simulink model "RobotSim_v0p1"  (R2025b)
settings: Solver=FixedStepAuto  StartTime=0.0  StopTime=99999  RelTol=1e-3
values from neighbouring files (symbols this model uses):
  maxSteeringVel = 0.5    [dogbot.m]
  maxVelocity = 0.5    [dogbot.m]
  rrtPath = rrtPlanner(startPose,goalPose,true,params)    [dogbot.m]    (also in rrtPlanner.m = [xvar,yvar,tvar]; rrtPlannerOld.m = [xvar',yvar',tvar'])
  stanleyGain = 0.5    [dogbot.m]
  wheelBase = 1.0    (= 1)    [dogbot.m]
  x0 = startPose(1)    [dogbot.m]
  y0 = startPose(2)    [dogbot.m]
undefined symbols (not defined in the file or in its folder): Bh, Bphi, Bva, Cg, Chi0, Cwind, h0, Hc, Phi0, Psi0, targetPose, Va0, Vc
libraries: ros2lib x2, instrumentlib x1
settings Model: PacingRate=158  Creator=benpo  LastModifiedBy=benpo
settings OptimizationCC: DefaultParameterBehavior=Inlined  EnhancedBackFolding=on  PassReuseOutputArgsAs=Individual arguments  ZeroExternalMemoryAtStartup=off  ZeroInternalMemoryAtStartup=off  MaxStackSize=64  OptimizeBlockOrder=speed  DifferentSizesBufferReuse=on  OptimizationCustomize=off  EfficientTunableParamExpr=on
settings DebuggingCC: ParameterTunabilityLossMsg=error
settings SFSimCC: MATLABDynamicMemAlloc=off
settings RTWCC: SystemTargetFile=ert.tlc  HardwareBoard=Robot Operating System 2 (ROS 2)  TLCOptions="-aInlineSetEventsForThisBaseRateFcn=TLC_FALSE -aSuppressMultiTaskScheduler=TLC_FALSE  -aRateBasedStepFcn=0"  TemplateMakefile=ert_default_tmf  Toolchain=Colcon Tools  TargetLang=C++  Description=Embedded Coder
settings CodeAppCC: ForceParamTrailComments=on  IgnoreCustomStorageClasses=off  OperatorAnnotations=on  SimulinkDataObjDesc=on  SFDataObjDesc=on  InsertBlockDesc=on
settings ERTTargetCC: ExtModeTransport=2.0  ExtModeStaticAlloc=on  ExtModeMexFile=ext_xcp  ExtModeIntrfLevel=Level2 - Open  RootIOFormat=Structure reference  CodeInterfacePackaging=C++ class

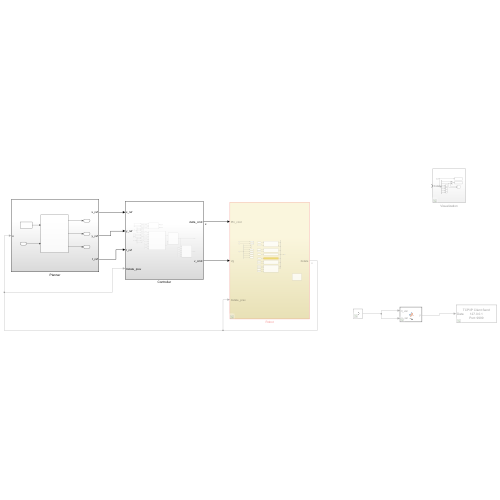
[thumbnail: Simulink's stored preview of the top-level diagram]
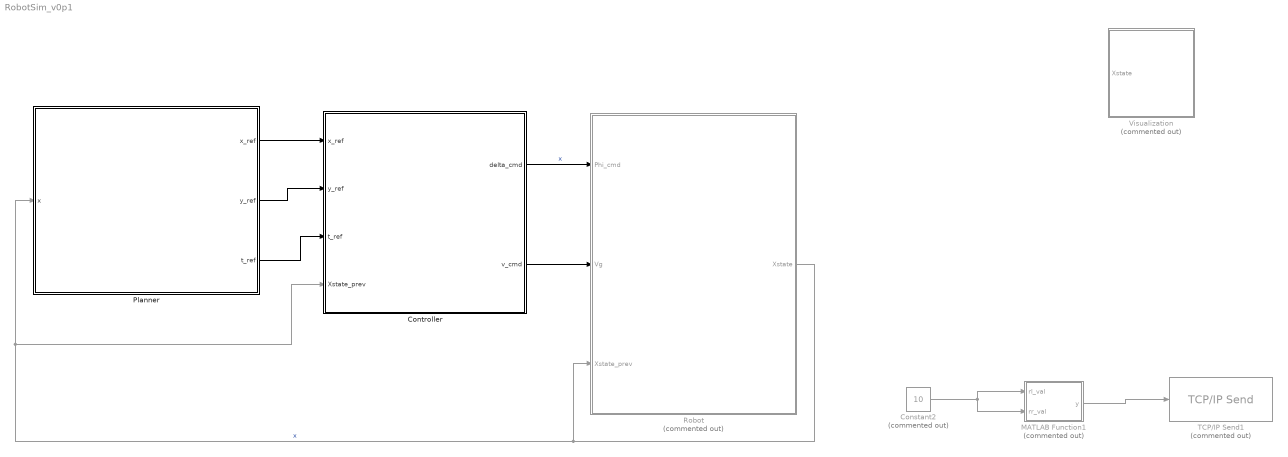
== system RobotSim_v0p1 ==
  Constant2 : Constant  Commented=on  Value=10
  Controller : Subsystem
  MATLAB Function1 : MATLAB Function  Commented=on  TreatAsAtomicUnit=on
  Planner : Subsystem
  Robot : Subsystem  Commented=on
  TCP/IP Send1 : instrumentlib/TCP//IP Send  Commented=on  Host=127.0.0.1  Port=9999  ByteOrder=big-endian  EnableBlockingMode=on  Timeout=10  TransferDelay=on  SimulateUsing=Interpreted execution
  Visualization : Subsystem  Commented=on
  wires:
  MATLAB Function1/1(y) -> TCP/IP Send1/1
  Constant2/1 -> MATLAB Function1/1(rl_val), MATLAB Function1/2(rr_val)
  Robot/1(Xstate) -> Robot/3(Xstate_prev), Controller/4(Xstate_prev), Planner/1(x)  "x"
  Controller/2(v_cmd) -> Robot/2(Vg)
  Controller/1(delta_cmd) -> Robot/1(Phi_cmd)  "x"
  Planner/1(x_ref) -> Controller/1(x_ref)
  Planner/2(y_ref) -> Controller/2(y_ref)
  Planner/3(t_ref) -> Controller/3(t_ref)

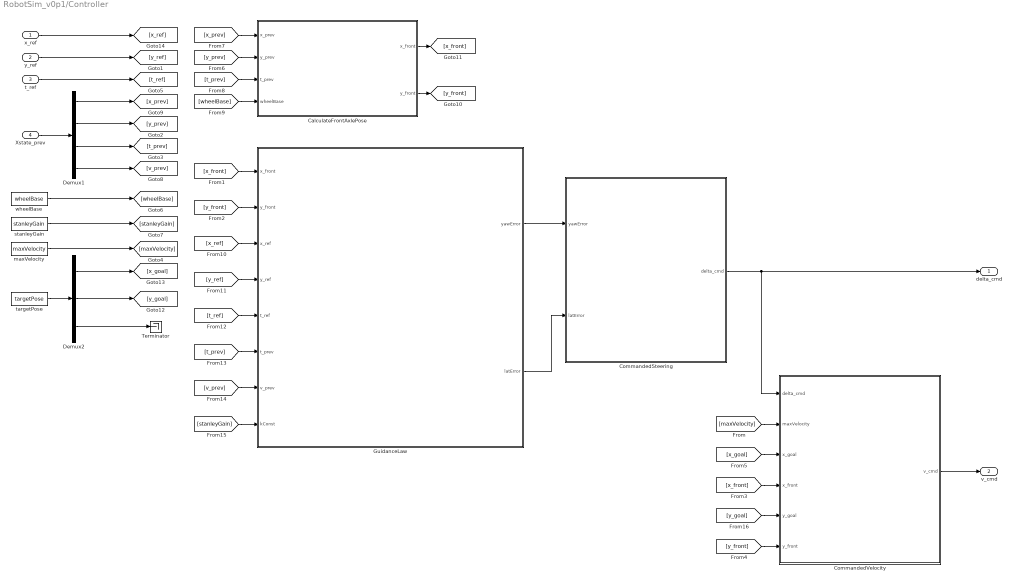
== system RobotSim_v0p1/Controller ==
  x_ref : Inport
  y_ref : Inport  Port=2
  t_ref : Inport  Port=3
  Xstate_prev : Inport  Port=4
  CalculateFrontAxlePose : Subsystem
  CommandedSteering : Subsystem
  CommandedVelocity : Subsystem
  Demux1 : Demux
  Demux2 : Demux  Outputs=3
  GuidanceLaw : Subsystem
  Terminator : Terminator
  maxVelocity : Constant  Value=maxVelocity
  stanleyGain : Constant  Value=stanleyGain
  targetPose : Constant  Value=targetPose
  wheelBase : Constant  Value=wheelBase
  delta_cmd : Outport
  v_cmd : Outport  Port=2
  wires:
  Xstate_prev/1 -> Demux1/1
  x_ref/1 -> [x_ref]
  Demux1/1 -> [x_prev]
  Demux1/3 -> [t_prev]
  Demux1/4 -> [v_prev]
  Demux1/2 -> [y_prev]
  y_ref/1 -> [y_ref]
  t_ref/1 -> [t_ref]
  [x_prev] -> CalculateFrontAxlePose/1(x_prev)
  [y_prev] -> CalculateFrontAxlePose/2(y_prev)
  [t_prev] -> CalculateFrontAxlePose/3(t_prev)
  wheelBase/1 -> [wheelBase]
  [wheelBase] -> CalculateFrontAxlePose/4(wheelBase)
  CalculateFrontAxlePose/2(y_front) -> [y_front]
  [x_ref] -> GuidanceLaw/3(x_ref)
  [y_ref] -> GuidanceLaw/4(y_ref)
  [t_ref] -> GuidanceLaw/5(t_ref)
  [t_prev] -> GuidanceLaw/6(t_prev)
  [v_prev] -> GuidanceLaw/7(v_prev)
  stanleyGain/1 -> [stanleyGain]
  [stanleyGain] -> GuidanceLaw/8(kConst)
  GuidanceLaw/2(latError) -> CommandedSteering/2(latError)
  GuidanceLaw/1(yawError) -> CommandedSteering/1(yawError)
  CommandedSteering/1(delta_cmd) -> CommandedVelocity/1(delta_cmd), delta_cmd/1
  maxVelocity/1 -> [maxVelocity]
  [maxVelocity] -> CommandedVelocity/2(maxVelocity)
  CommandedVelocity/1(v_cmd) -> v_cmd/1
  CalculateFrontAxlePose/1(x_front) -> [x_front]
  [x_front] -> GuidanceLaw/1(x_front)
  [y_front] -> GuidanceLaw/2(y_front)
  [y_front] -> CommandedVelocity/6(y_front)
  [x_front] -> CommandedVelocity/4(x_front)
  targetPose/1 -> Demux2/1
  Demux2/1 -> [x_goal]
  Demux2/2 -> [y_goal]
  Demux2/3 -> Terminator/1
  [x_goal] -> CommandedVelocity/3(x_goal)
  [y_goal] -> CommandedVelocity/5(y_goal)

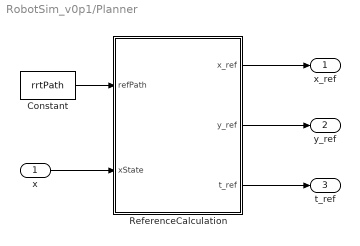
== system RobotSim_v0p1/Planner ==
  x : Inport
  Constant : Constant  Value=rrtPath
  ReferenceCalculation : MATLAB Function  TreatAsAtomicUnit=on
  x_ref : Outport
  y_ref : Outport  Port=2
  t_ref : Outport  Port=3
  wires:
  ReferenceCalculation/3(t_ref) -> t_ref/1
  Constant/1 -> ReferenceCalculation/1(refPath)
  ReferenceCalculation/1(x_ref) -> x_ref/1
  ReferenceCalculation/2(y_ref) -> y_ref/1
  x/1 -> ReferenceCalculation/2(xState)

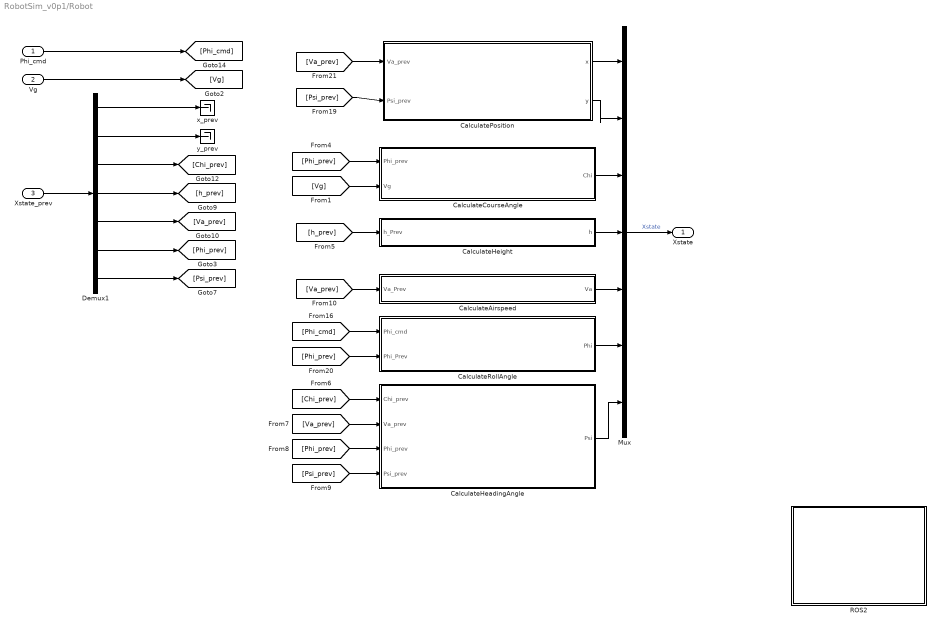
== system RobotSim_v0p1/Robot ==
  Phi_cmd : Inport
  Vg : Inport  Port=2
  Xstate_prev : Inport  Port=3
  CalculateAirspeed : Subsystem
  CalculateCourseAngle : Subsystem
  CalculateHeadingAngle : Subsystem
  CalculateHeight : Subsystem
  CalculatePosition : Subsystem
  CalculateRollAngle : Subsystem
  Demux1 : Demux  Outputs=7
  Mux : Mux  Inputs=7
  ROS2 : Subsystem
  x_prev : Terminator
  y_prev : Terminator
  Xstate : Outport
  wires:
  Phi_cmd/1 -> [Phi_cmd]
  [Phi_cmd] -> CalculateRollAngle/1(Phi_cmd)
  CalculateRollAngle/1(Phi) -> Mux/6
  [Phi_prev] -> CalculateRollAngle/2(Phi_Prev)
  Xstate_prev/1 -> Demux1/1
  Demux1/6 -> [Phi_prev]
  Demux1/7 -> [Psi_prev]
  Demux1/5 -> [Va_prev]
  Demux1/4 -> [h_prev]
  Demux1/3 -> [Chi_prev]
  CalculatePosition/1(x) -> Mux/1
  CalculatePosition/2(y) -> Mux/2
  [Va_prev] -> CalculatePosition/1(Va_prev)
  [Psi_prev] -> CalculatePosition/2(Psi_prev)
  Mux/1 -> Xstate/1  "Xstate"
  [Phi_prev] -> CalculateCourseAngle/1(Phi_prev)
  CalculateCourseAngle/1(Chi) -> Mux/3
  [Vg] -> CalculateCourseAngle/2(Vg)
  CalculateHeight/1(h) -> Mux/4
  [h_prev] -> CalculateHeight/1(h_Prev)
  CalculateHeadingAngle/1(Psi) -> Mux/7
  [Chi_prev] -> CalculateHeadingAngle/1(Chi_prev)
  [Va_prev] -> CalculateHeadingAngle/2(Va_prev)
  [Phi_prev] -> CalculateHeadingAngle/3(Phi_prev)
  [Psi_prev] -> CalculateHeadingAngle/4(Psi_prev)
  CalculateAirspeed/1(Va) -> Mux/5
  [Va_prev] -> CalculateAirspeed/1(Va_Prev)
  Demux1/1 -> x_prev/1
  Demux1/2 -> y_prev/1
  Vg/1 -> [Vg]

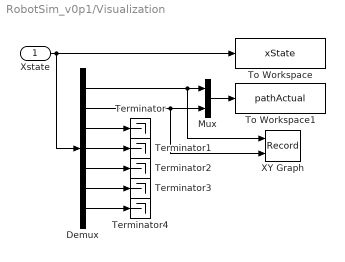
== system RobotSim_v0p1/Visualization ==
  Xstate : Inport
  Demux : Demux  Outputs=7
  Mux : Mux  Inputs=2
  Terminator{,1..4} (5 alike) : Terminator
  To Workspace : ToWorkspace  VariableName=xState  SampleTime=-1
  To Workspace1 : ToWorkspace  VariableName=pathActual  SampleTime=-1
  XY Graph : Record  NumPorts=2.0  FileSettingsInternal="{\"entries\":[{\"content\":{\"excelSettings\":{\"content\":{},\"type\":\"Streamout.ExcelSettings\"},\"parquetSettings\":{\"content\":{},\"type\":\"Streamout.ParquetSettings\"}},\"type\":\"Streamout.FileSettingStorage\",\"uuid\":\"\"}],\"packageUris\":[\"http:\\/\\/schema.mathworks.com\\/mf0\\/streamout_blocks\\/R2020a\"],\"version\":\"1.0\"}"  FrameSettings=[0, 0]  Layout=[1 1]  SignalsInternal="{\"entries\":[{\"content\":{\"signals\":[{\"content\":{\"blockPath\":[],\"dimensions\":[1],\"domain\":\"\",\"lineColor\":\"#a2142f\",\"plots\":[ 1 ],\"port\":1,\"signalID\":1,\"signalName\":\"Demux:1\"},\"type\":\"RecordBlkView.Signal\",\"uuid\":\"\"},{\"content\":{\"blockPath\":[],\"dimensions\":[1],\"domain\":\"\",\"lineColor\":\"#139fff\",\"plots\":[ 1 ],\"port\":2,\"signalID\":2,\"signalName\":\"Demux:2\"},\"type\":\"RecordBlkView.Signal\",\"uuid\":\"\"}]},\"type\":\"RecordBlkView.InputSignals\",\"uuid\":\"\"}],\"packageUris\":[\"http:\\/\\/schema.mathworks.com\\/mf0\\/streamout_blocks\\/R2020a\"],\"version\":\"1.0\"}"  VisualizationBindings="{\"xyplotplugin\":{\"info\":[{\"series\":[{\"bindingParametersList\":[{\"parameter\":\"X-Axis\",\"signalID\":1,\"signalName\":\"Demux:1\"},{\"parameter\":\"Y-Axis\",\"signalID\":2,\"signalName\":\"Demux:2\"}],\"seriesID\":0}],\"subplotID\":1}]}}"  CompatibilityTag=XY
  wires:
  Xstate/1 -> Demux/1, To Workspace/1
  Mux/1 -> To Workspace1/1
  Demux/1 -> XY Graph/1, Mux/1
  Demux/2 -> XY Graph/2, Mux/2
  Demux/3 -> Terminator/1
  Demux/4 -> Terminator1/1
  Demux/5 -> Terminator2/1
  Demux/6 -> Terminator3/1
  Demux/7 -> Terminator4/1

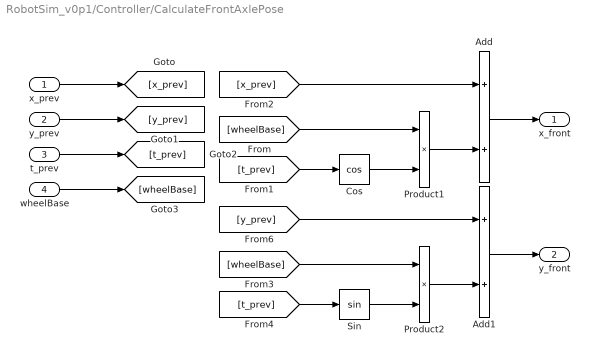
== system RobotSim_v0p1/Controller/CalculateFrontAxlePose ==
  x_prev : Inport
  y_prev : Inport  Port=2
  t_prev : Inport  Port=3
  wheelBase : Inport  Port=4
  Add : Sum
  Add1 : Sum
  Cos : Trigonometry  Operator=cos
  Product1 : Product
  Product2 : Product
  Sin : Trigonometry
  x_front : Outport
  y_front : Outport  Port=2
  wires:
  y_prev/1 -> [y_prev]
  x_prev/1 -> [x_prev]
  t_prev/1 -> [t_prev]
  wheelBase/1 -> [wheelBase]
  Add/1 -> x_front/1
  Product1/1 -> Add/2
  Cos/1 -> Product1/2
  [wheelBase] -> Product1/1
  [t_prev] -> Cos/1
  [x_prev] -> Add/1
  [y_prev] -> Add1/1
  [t_prev] -> Sin/1
  [wheelBase] -> Product2/1
  Sin/1 -> Product2/2
  Product2/1 -> Add1/2
  Add1/1 -> y_front/1

== system RobotSim_v0p1/Controller/CommandedSteering ==
  yawError : Inport
  latError : Inport  Port=2
  Add : Sum
  Saturation : Saturate  UpperLimit=maxSteeringVel  LowerLimit=-maxSteeringVel
      settings: AttributesFormatString=[%<LowerLimit>,%<UpperLimit>]
  delta_cmd : Outport
  wires:
  latError/1 -> Add/2
  yawError/1 -> Add/1
  Saturation/1 -> delta_cmd/1
  Add/1 -> Saturation/1

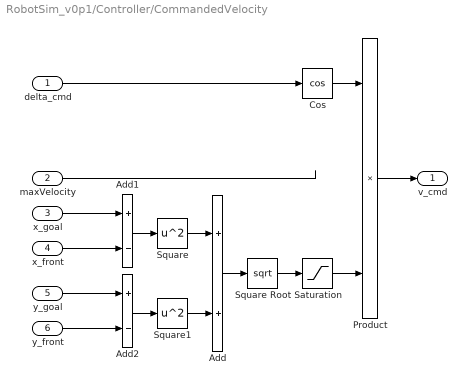
== system RobotSim_v0p1/Controller/CommandedVelocity ==
  delta_cmd : Inport
  maxVelocity : Inport  Port=2
  x_goal : Inport  Port=3
  x_front : Inport  Port=4
  y_goal : Inport  Port=5
  y_front : Inport  Port=6
  Add : Sum
  Add1 : Sum  Inputs=+-
  Add2 : Sum  Inputs=+-
  Cos : Trigonometry  Operator=cos
  Product : Product  Inputs=3
  Saturation : Saturate  UpperLimit=1  LowerLimit=0
      settings: AttributesFormatString=[%<LowerLimit>,%<UpperLimit>]
  Square : Math  Operator=square
  Square Root : Sqrt
  Square1 : Math  Operator=square
  v_cmd : Outport
  wires:
  Product/1 -> v_cmd/1
  delta_cmd/1 -> Cos/1
  maxVelocity/1 -> ?
  Cos/1 -> Product/1
  Square/1 -> Add/1
  Square1/1 -> Add/2
  Add/1 -> Square Root/1
  Add1/1 -> Square/1
  Add2/1 -> Square1/1
  x_front/1 -> Add1/2
  x_goal/1 -> Add1/1
  y_goal/1 -> Add2/1
  y_front/1 -> Add2/2
  Square Root/1 -> Saturation/1
  Saturation/1 -> Product/3

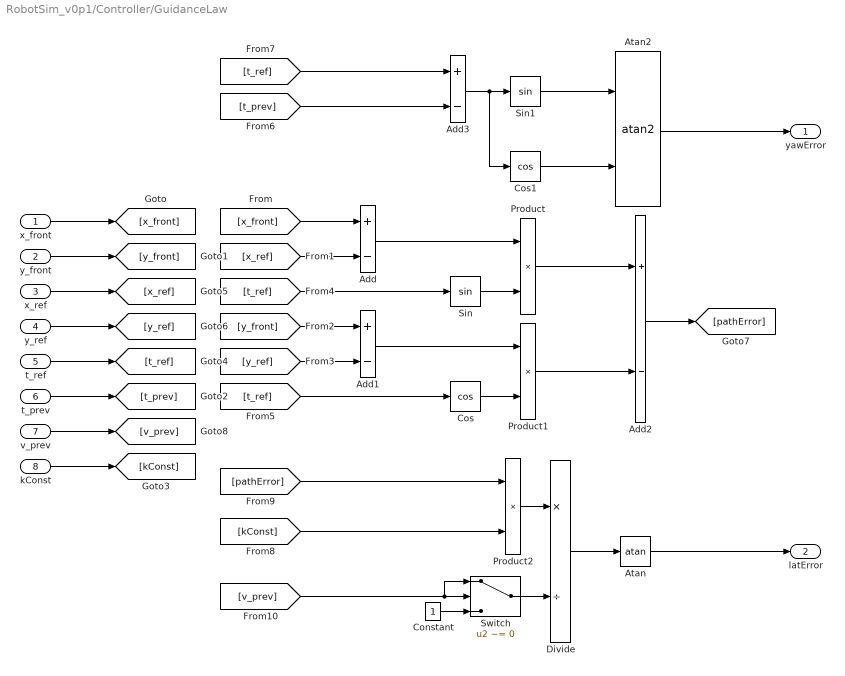
== system RobotSim_v0p1/Controller/GuidanceLaw ==
  x_front : Inport
  y_front : Inport  Port=2
  x_ref : Inport  Port=3
  y_ref : Inport  Port=4
  t_ref : Inport  Port=5
  t_prev : Inport  Port=6
  v_prev : Inport  Port=7
  kConst : Inport  Port=8
  Add{,1..3} (4 alike) : Sum  Inputs=+-
  Atan : Trigonometry  Operator=atan
  Atan2 : Trigonometry  Operator=atan2
  Constant : Constant
  Cos : Trigonometry  Operator=cos
  Cos1 : Trigonometry  Operator=cos
  Divide : Product  Inputs=*/
  Product : Product
  Product1 : Product
  Product2 : Product
  Sin : Trigonometry
  Sin1 : Trigonometry
  Switch : Switch  Criteria=u2 ~= 0  SaturateOnIntegerOverflow=off  InputSameDT=off
  yawError : Outport
  latError : Outport  Port=2
  wires:
  kConst/1 -> [kConst]
  t_prev/1 -> [t_prev]
  x_front/1 -> [x_front]
  y_front/1 -> [y_front]
  t_ref/1 -> [t_ref]
  Add2/1 -> [pathError]
  y_ref/1 -> [y_ref]
  x_ref/1 -> [x_ref]
  [x_front] -> Add/1
  [x_ref] -> Add/2
  Product/1 -> Add2/1
  Add/1 -> Product/1
  Sin/1 -> Product/2
  [t_ref] -> Sin/1
  [t_ref] -> Cos/1
  Cos/1 -> Product1/2
  Add1/1 -> Product1/1
  Product1/1 -> Add2/2
  [y_ref] -> Add1/2
  [y_front] -> Add1/1
  Atan2/1 -> yawError/1
  Sin1/1 -> Atan2/1
  Cos1/1 -> Atan2/2
  Add3/1 -> Cos1/1, Sin1/1
  [t_prev] -> Add3/2
  [t_ref] -> Add3/1
  Atan/1 -> latError/1
  [kConst] -> Product2/2
  [pathError] -> Product2/1
  Product2/1 -> Divide/1
  v_prev/1 -> [v_prev]
  Switch/1 -> Divide/2
  [v_prev] -> Switch/1, Switch/2
  Constant/1 -> Switch/3
  Divide/1 -> Atan/1

== system RobotSim_v0p1/Robot/CalculateAirspeed ==
  Va_Prev : Inport
  Add5 : Sum  Inputs=+-
  Gain : Gain  Gain=Bva
  Integrator7 : Integrator  InitialCondition=Va0
      settings: AttributesFormatString=Initial Condition: %<InitialCondition>
  Vc : Constant  Value=Vc
  Va : Outport
  wires:
  Add5/1 -> Gain/1
  Gain/1 -> Integrator7/1  "Va_dot"
  Vc/1 -> Add5/1
  Va_Prev/1 -> Add5/2
  Integrator7/1 -> Va/1  "Va"

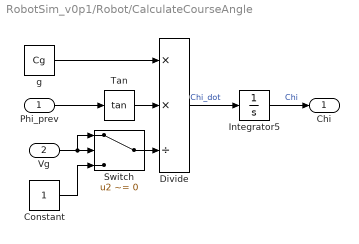
== system RobotSim_v0p1/Robot/CalculateCourseAngle ==
  Phi_prev : Inport
  Vg : Inport  Port=2
  Constant : Constant
  Divide : Product  Inputs=**/
  Integrator5 : Integrator  InitialCondition=Chi0
      settings: AttributesFormatString=Initial Condition: %<InitialCondition>
  Switch : Switch  Criteria=u2 ~= 0  SaturateOnIntegerOverflow=off  InputSameDT=off
  Tan : Trigonometry  Operator=tan
  g : Constant  Value=Cg
  Chi : Outport
  wires:
  Tan/1 -> Divide/2
  Divide/1 -> Integrator5/1  "Chi_dot"
  Phi_prev/1 -> Tan/1
  Integrator5/1 -> Chi/1  "Chi"
  g/1 -> Divide/1
  Switch/1 -> Divide/3
  Vg/1 -> Switch/2, Switch/1
  Constant/1 -> Switch/3

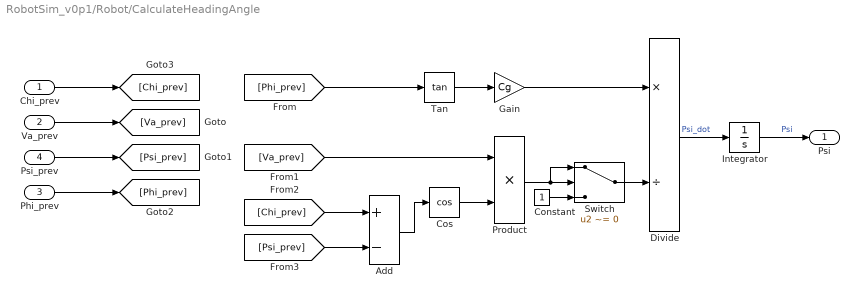
== system RobotSim_v0p1/Robot/CalculateHeadingAngle ==
  Chi_prev : Inport
  Va_prev : Inport  Port=2
  Phi_prev : Inport  Port=3
  Psi_prev : Inport  Port=4
  Add : Sum  Inputs=+-
  Constant : Constant
  Cos : Trigonometry  Operator=cos
  Divide : Product  Inputs=*/
  Gain : Gain  Gain=Cg
  Integrator : Integrator  InitialCondition=Psi0
      settings: AttributesFormatString=Initial Condition: %<InitialCondition>
  Product : Product
  Switch : Switch  Criteria=u2 ~= 0  SaturateOnIntegerOverflow=off  InputSameDT=off
  Tan : Trigonometry  Operator=tan
  Psi : Outport
  wires:
  Psi_prev/1 -> [Psi_prev]
  Va_prev/1 -> [Va_prev]
  Integrator/1 -> Psi/1  "Psi"
  Divide/1 -> Integrator/1  "Psi_dot"
  Phi_prev/1 -> [Phi_prev]
  Chi_prev/1 -> [Chi_prev]
  [Phi_prev] -> Tan/1
  Gain/1 -> Divide/1
  Tan/1 -> Gain/1
  Product/1 -> Switch/1, Switch/2
  Cos/1 -> Product/2
  [Va_prev] -> Product/1
  Add/1 -> Cos/1
  [Chi_prev] -> Add/1
  [Psi_prev] -> Add/2
  Switch/1 -> Divide/2
  Constant/1 -> Switch/3

== system RobotSim_v0p1/Robot/CalculateHeight ==
  h_Prev : Inport
  Add5 : Sum  Inputs=+-
  Bh1 : Constant  Value=Hc
  Gain : Gain  Gain=Bh
  Integrator7 : Integrator  InitialCondition=h0
      settings: AttributesFormatString=Initial Condition: %<InitialCondition>
  h : Outport
  wires:
  Integrator7/1 -> h/1  "h"
  h_Prev/1 -> Add5/2
  Bh1/1 -> Add5/1
  Gain/1 -> Integrator7/1  "h_dot"
  Add5/1 -> Gain/1

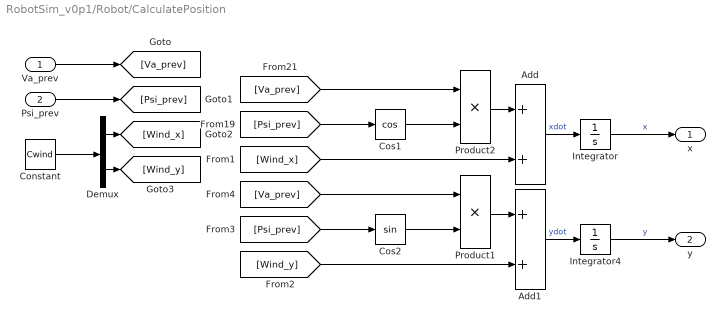
== system RobotSim_v0p1/Robot/CalculatePosition ==
  Va_prev : Inport
  Psi_prev : Inport  Port=2
  Add : Sum
  Add1 : Sum
  Constant : Constant  Value=Cwind
  Cos1 : Trigonometry  Operator=cos
  Cos2 : Trigonometry
  Demux : Demux  Outputs=2
  Integrator : Integrator  InitialCondition=x0
      settings: AttributesFormatString=Initial Condition: %<InitialCondition>
  Integrator4 : Integrator  InitialCondition=y0
      settings: AttributesFormatString=Initial Condition: %<InitialCondition>
  Product1 : Product
  Product2 : Product
  x : Outport
  y : Outport  Port=2
  wires:
  Product2/1 -> Add/1
  Add1/1 -> Integrator4/1  "ydot"
  Add/1 -> Integrator/1  "xdot"
  Integrator/1 -> x/1  "x"
  Cos1/1 -> Product2/2
  Integrator4/1 -> y/1  "y"
  [Va_prev] -> Product2/1
  [Psi_prev] -> Cos1/1
  Va_prev/1 -> [Va_prev]
  Psi_prev/1 -> [Psi_prev]
  Constant/1 -> Demux/1
  Demux/1 -> [Wind_x]
  Demux/2 -> [Wind_y]
  [Wind_x] -> Add/2
  [Wind_y] -> Add1/2
  [Psi_prev] -> Cos2/1
  [Va_prev] -> Product1/1
  Cos2/1 -> Product1/2
  Product1/1 -> Add1/1

== system RobotSim_v0p1/Robot/CalculateRollAngle ==
  Phi_cmd : Inport
  Phi_Prev : Inport  Port=2
  Add5 : Sum  Inputs=+-
  Gain : Gain  Gain=Bphi
  Integrator7 : Integrator  InitialCondition=Phi0
      settings: AttributesFormatString=Initial Condition: %<InitialCondition>
  Phi : Outport
  wires:
  Add5/1 -> Gain/1
  Gain/1 -> Integrator7/1  "Phi_dot"
  Phi_cmd/1 -> Add5/1
  Phi_Prev/1 -> Add5/2
  Integrator7/1 -> Phi/1  "Phi"

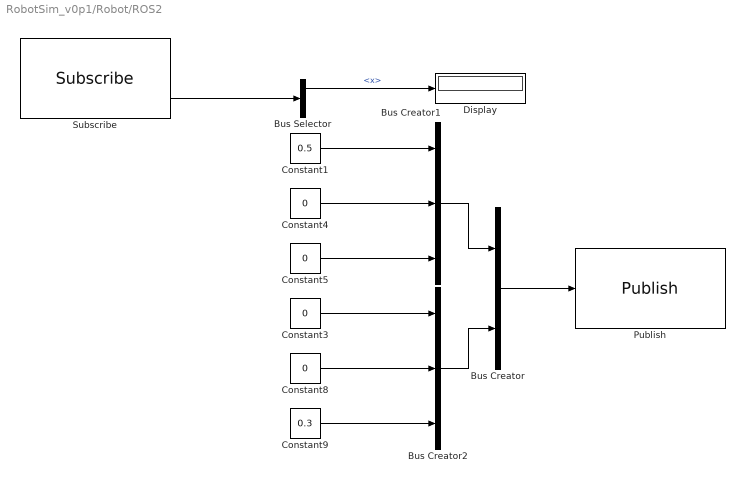
== system RobotSim_v0p1/Robot/ROS2 ==
  Bus Creator : BusCreator  Inputs=2  OutDataTypeStr=Bus: SL_Bus_geometry_msgs_Twist  NonVirtualBus=on
      settings: InheritFromInputs=off
  Bus Creator1 : BusCreator  Inputs=3  OutDataTypeStr=Bus: SL_Bus_geometry_msgs_Vector3  NonVirtualBus=on
      settings: InheritFromInputs=off
  Bus Creator2 : BusCreator  Inputs=3  OutDataTypeStr=Bus: SL_Bus_geometry_msgs_Vector3  NonVirtualBus=on
      settings: InheritFromInputs=off
  Bus Selector : BusSelector  OutputSignals=pose.pose.position.x,pose.pose.position.y,pose.pose.orientation.x
  Constant1 : Constant  Value=0.5
  Constant{3..5,8} (4 alike) : Constant  Value=0
  Constant9 : Constant  Value=0.3
  Display : Display
  Publish : ros2lib/Publish  topicSource=Specify your own  topic=/model/dog_bot/cmd_vel  messageType=geometry_msgs/Twist  QOSHistory=Keep last  QOSDepth=10  QOSReliability=Reliable  QOSDurability=Volatile  QOSDeadline=Inf  QOSLifespan=Inf  QOSLiveliness=Automatic  QOSLeaseDuration=Inf  QOSAvoidROSNamespaceConventions=off
  Subscribe : ros2lib/Subscribe  topicSource=Specify your own  topic=/model/dog_bot/odometry  messageType=nav_msgs/Odometry  sampleTime=-1  QOSHistory=Keep last  QOSDepth=10  QOSReliability=Reliable  QOSDurability=Volatile  QOSDeadline=Inf  QOSLifespan=Inf  QOSLiveliness=Automatic  QOSLeaseDuration=Inf  QOSAvoidROSNamespaceConventions=off
  wires:
  Bus Creator2/1 -> Bus Creator/2
  Constant5/1 -> Bus Creator1/3
  Bus Selector/1 -> Display/1  "<x>"
  Constant1/1 -> Bus Creator1/1
  Constant8/1 -> Bus Creator2/2
  Constant3/1 -> Bus Creator2/1
  Bus Creator/1 -> Publish/1
  Constant9/1 -> Bus Creator2/3
  Bus Creator1/1 -> Bus Creator/1
  Constant4/1 -> Bus Creator1/2
  Subscribe/2 -> Bus Selector/1

== matlab function RobotSim_v0p1/MATLAB Function1 ==
  data: rl_val input; y output uint8 size=[1 64]; rr_val input
function y = fcn(rl_val, rr_val)
    % 1. Create a fixed-size buffer of 64 bytes (larger for two commands)
    y = repmat(uint8(' '), 1, 64); 
    
    % 2. Combine commands with a semicolon
    % Example: 'rl_drive_j 5.0;rr_drive_j 5.0'
    str = [ 'rl_drive_j ', num2str(round(rl_val*100)/100), ...
            ';rr_drive_j ', num2str(round(rr_val*100)/100) ];
    
    bytes = uint8(str);
    len = min(length(bytes), 64);
    y(1:len) = bytes(1:len);
end

== matlab function RobotSim_v0p1/Planner/ReferenceCalculation ==
  settings: updateMethod=DISCRETE
  data: refPath input; x_ref output; xState input; y_ref output; t_ref output
function [x_ref,y_ref,t_ref] = getTrackingTarget(refPath,xState)
% xstate = [x,y,theta,vel]
persistent lastIdx;
if isempty(lastIdx)
    lastIdx = 1;
end % if

% Params
useWindow = 50; % current path is 500, so old value of 250 is too large
L0 = 1.0;
kv = 0.4;

pathX = refPath(:,1);
pathY = refPath(:,2);
pathT = refPath(:,3); % get tangent
N = size(refPath,1);

x = xState(1);
y = xState(2);
v = xState(4);

% find nearest point
i0 = lastIdx;
i1 = min(N,i0+useWindow);

dx = pathX(i0:i1)-x;
dy = pathY(i0:i1)-y;
[~,wayptIdx] = min(dx.^2+dy.^2);
i_near = i0+wayptIdx-1;
lastIdx = i_near;

% calc params
Ld = max(1,min(L0+kv*abs(v),2.0));

% lookahead target
i_target = i_near;
dist_acc = 0;
while i_target < N && dist_acc < Ld
    ddx = pathX(i_target+1) - pathX(i_target);
    ddy = pathY(i_target+1) - pathY(i_target);
    dist_acc = dist_acc + sqrt(ddx^2 + ddy^2);
    i_target = i_target+1;
end % while
x_ref = pathX(i_target);
y_ref = pathY(i_target);
t_ref = pathT(i_target);

end % func
